simulink library "Lib_HeatXfer_1DtransconductionFDE_TMATS_org"  (Simulink 10.0)
settings: Solver=ode45  StartTime=0.0  StopTime=10.0  RelTol=1e-3  EnableMultiTasking=on
Description:
  | Thomas Modules
settings Model: Creator=jwchapm2  LastModifiedBy=annonymous

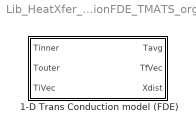
== system Lib_HeatXfer_1DtransconductionFDE_TMATS_org ==
  1-D Trans Conduction model (FDE) : Subsystem  mask(T-MATS: 1-D Trans Cond Model(FDE) Block){dt_M=4, Nod_M=4, w_M=4, h_M=1, k_M=2, rho_M=3, c_M=4, BlkNm_M=double(gcb)}
      mask prompts: dt_M "dt_M - Time Step"; Nod_M "Nod_M - Numer of Nodes"; w_M "w_M - Plate Width"; h_M "h_M - convection heat transfer coefficient"; k_M "k_M - thermal conductivity"; rho_M "rho_M - mass density"; c_M "c_M - specific heat"; BlkNm_M "BlkNm_M - Block Name"
      mask help:
      | This function models the transient conduction of a plate with fluid on either side via the finite difference method (explicit).
      |
      | Export values are calculated based on a single time step. If additional dynamic behavior is required a simulink memory block may be used to update the temperature initial conditions.
      mask Help: web(which('HeatXfer_TMATS_1DTCondFDE.html'),'-helpbrowser')

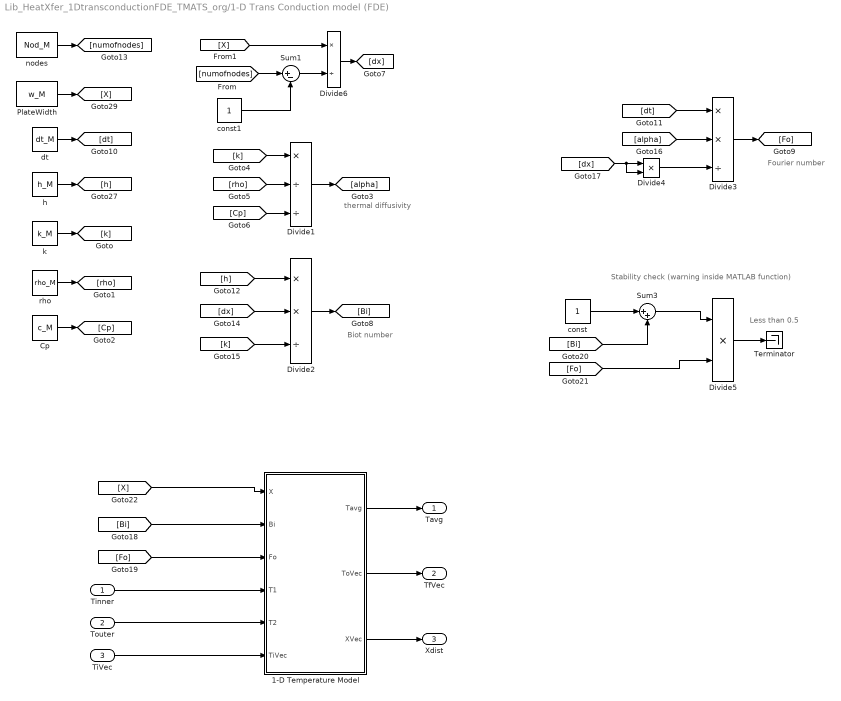
== system Lib_HeatXfer_1DtransconductionFDE_TMATS_org/1-D Trans Conduction model (FDE) ==
  note: Stability check (warning inside MATLAB function)
  note: Less than 0.5
  note: Fourier number
  note: Biot number
  note: thermal diffusivity
  Tinner : Inport
  Touter : Inport  Port=2
  TiVec : Inport  Port=3
  1-D Temperature Model : MATLAB Function  TreatAsAtomicUnit=on
  Cp : Constant  Value=c_M
  Divide1 : Product  Inputs=*//
  Divide2 : Product  Inputs=**/
  Divide3 : Product  Inputs=**/
  Divide4 : Product  Inputs=**
  Divide5 : Product  Inputs=**
  Divide6 : Product  Inputs=*/
  PlateWidth : Constant  Value=w_M
  Sum1 : Sum  Inputs=|+-
  Sum3 : Sum  Inputs=|++
  Terminator : Terminator
  const : Constant
  const1 : Constant
  dt : Constant  Value=dt_M
  h : Constant  Value=h_M
  k : Constant  Value=k_M
  nodes : Constant  Value=Nod_M
  rho : Constant  Value=rho_M
  Tavg : Outport
  TfVec : Outport  Port=2
  Xdist : Outport  Port=3
  wires:
  Divide6/1 -> [dx]
  [X] -> Divide6/1
  Sum1/1 -> Divide6/2
  const1/1 -> Sum1/2
  [numofnodes] -> Sum1/1
  PlateWidth/1 -> [X]
  Touter/1 -> 1-D Temperature Model/5(T2)
  Tinner/1 -> 1-D Temperature Model/4(T1)
  TiVec/1 -> 1-D Temperature Model/6(TiVec)
  1-D Temperature Model/1(Tavg) -> Tavg/1
  1-D Temperature Model/2(ToVec) -> TfVec/1
  1-D Temperature Model/3(XVec) -> Xdist/1
  h/1 -> [h]
  [dt] -> Divide3/1
  [alpha] -> Divide3/2
  dt/1 -> [dt]
  [dx] -> Divide4/2, Divide4/1
  nodes/1 -> [numofnodes]
  [dx] -> Divide2/2
  [k] -> Divide1/1
  Divide3/1 -> [Fo]
  [k] -> Divide2/3
  Divide2/1 -> [Bi]
  Divide1/1 -> [alpha]
  Cp/1 -> [Cp]
  [Bi] -> 1-D Temperature Model/2(Bi)
  rho/1 -> [rho]
  k/1 -> [k]
  [h] -> Divide2/1
  const/1 -> Sum3/1
  Divide4/1 -> Divide3/3
  [rho] -> Divide1/2
  [Cp] -> Divide1/3
  Divide5/1 -> Terminator/1
  [Bi] -> Sum3/2
  [Fo] -> Divide5/2
  [Fo] -> 1-D Temperature Model/3(Fo)
  [X] -> 1-D Temperature Model/1(X)
  Sum3/1 -> Divide5/1

== matlab function 1-D Trans Conduction model (FDE)/1-D Temperature Model ==
  data: X input double; Bi input double; Tavg output double; Fo input double; T1 input double; T2 input double; TiVec input double; ToVec output double; XVec output double; Nod_M parameter double; BlkNm_M parameter double
function [Tavg, ToVec, XVec] = fcn(X, Bi, Fo, T1, T2, TiVec, Nod_M, BlkNm_M)
% Written by Jeffyres Chapman
%
% This function models the heat transfer of a plate with fluid on either 
% side via the finite difference method (explicit)
% Per "Fundamentals of Heat and Mass Transfer" 5th edition, Incropera and
% DeWitt, section 5.9
%               |            |
%               |            |
%               |            |
%    Fluid 1    |   Solid    |  Fluid 2
%               |            |
%               |            |
%               |            |
%               |            |
%
% Inputs
% T1 - Inner temperature
% T2 - outer temperature
% TiVec - initial temperature states
% X - width of plate
% nodes - number of nodes
% Fo - Fourier number = alpha * delta_t/ (delta_x)^2
% Bi - Biot number = h * delta_x/k
% Nod_M - number of Nodes and States (located within Mask)
% BlkNm_M - Block name (located within Mask)
%
% Outputs
% XVec - vector of distances from inner -> outer
% ToVec - output temperature vector
% Tavg - Average Temperature

%Initialize
States = Nod_M;
XVec = zeros(States,1);
Nw = XVec;
ToVec = TiVec;
dx = X/(States - 1);
Tavg = 1;

% check to determine if all states are stable
if Fo > 0.5 
    disp('Error in %c, Fo > 0.5, input properties not appropriate for modeling method', BlkNm_M);
elseif Fo*(1+Bi) > 0.5
    disp(['Error in block ', BlkNm_M,', Fo*(1+Bi) > 0.5 , input properties not appropriate for modeling method']);
else
    % Calculate each updated node state
    ToVec(1) = 2* Fo * (TiVec(2) + Bi*T1)+ (1 - 2*Fo - 2*Bi*Fo)* TiVec(1);
    XVec(1) = 0;
    Nw(1) = dx/2;
    for i = 2: States -1
        ToVec(i) = Fo * (TiVec(i+1) + TiVec(i-1)) + (1 - 2*Fo)*TiVec(i);
        XVec(i) = XVec(i-1) + dx;
        Nw(i) = dx;
    end
    ToVec(States) = 2* Fo * (TiVec(States - 1) + Bi*T2)+ (1 - 2*Fo - 2*Bi*Fo)* TiVec(States);
    XVec(States) = XVec(States -1) + dx;
    Nw(States) = dx/2;

    Tavg = sum(ToVec.*Nw)/sum(Nw);
end
